simulink model "AariaHIABR2017a"  (R2017a)
settings: Solver=VariableStepAuto  StartTime=0.0  StopTime=inf  FixedStep=0.1  RelTol=1e-3  EnableMultiTasking=on
model workspace (MATLAB code in the model file):
  | my_a =1;
undefined symbols (not defined in the file or in its folder): AARIAENV, AARIAMAN, AARIASEN, Camera, sensor, Source_TS, X, Y, Z
libraries: sm_lib x347, nesl_utility x194, dspmathops x74, simulink x72, vrlib x2, powerlib_meascontrol x1, aerolibanimutils x1, aerolibutil x1
(part 6 of 9)

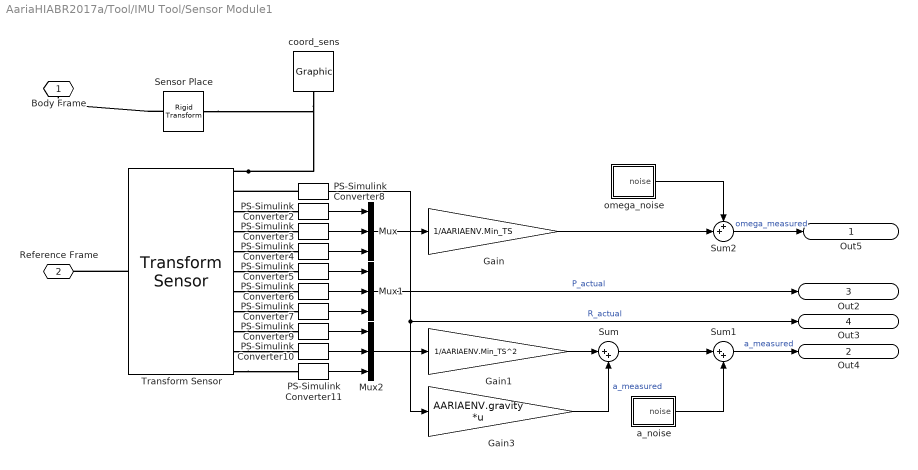
== system AariaHIABR2017a/Tool/IMU Tool/Sensor Module1 ==
  Gain : Gain  Gain=1/AARIAENV.Min_TS
  Gain1 : Gain  Gain=1/AARIAENV.Min_TS^2
  Gain3 : Gain  Gain=AARIAENV.gravity  Multiplication=Matrix(K*u)
  Mux : Mux  Inputs=3
  Mux1 : Mux  Inputs=3
  Mux2 : Mux  Inputs=3
  PS-Simulink Converter{5..11} (7 alike) : nesl_utility/PS-Simulink Converter  PhysicalDomain=network_engine_domain  SubClassName=ps_output  LeftPortType=input  RightPortType=output  PseudoPeriodic=off  Frequencies=[]  Unit=1  AffineConversion=off
  PS-Simulink Converter2 : nesl_utility/PS-Simulink Converter  PhysicalDomain=network_engine_domain  SubClassName=ps_output  LeftPortType=input  RightPortType=output  PseudoPeriodic=off  Frequencies=[]  Unit=rad/s  AffineConversion=off
  PS-Simulink Converter3 : nesl_utility/PS-Simulink Converter  PhysicalDomain=network_engine_domain  SubClassName=ps_output  LeftPortType=input  RightPortType=output  PseudoPeriodic=off  Frequencies=[]  Unit=rad/s  AffineConversion=off
  PS-Simulink Converter4 : nesl_utility/PS-Simulink Converter  PhysicalDomain=network_engine_domain  SubClassName=ps_output  LeftPortType=input  RightPortType=output  PseudoPeriodic=off  Frequencies=[]  Unit=rad/s  AffineConversion=off
  Sensor Place : sm_lib/Frames and Transforms/Rigid Transform  TranslationMethod=Cartesian  TranslationStandardOffset=0  TranslationLengthUnit=m  TranslationStandardAxis=+Z  TranslationCartesianOffset=AARIAMAN.L(nL).S(nS).pose_p  TranslationROffset=0  TranslationROffsetUnits=m  TranslationZOffset=0  TranslationZOffsetUnits=m  TranslationThetaOffset=0  TranslationThetaOffsetUnits=deg  RotationMethod=RotationMatrix  RotationAngleUnits=deg  RotationStandardAxis=+Z  RotationAngle=0.0  RotationArbitraryAxis=[0 0 1]  FollAlignAxisA=+X  BaseAlignAxisA=+Y  FollAlignAxisB=+Y  BaseAlignAxisB=+Z  RotationSequenceAxes=FollowerAxes  RotationSequence=XYX  RotationSequenceAngles=[0 0 0]  RotationSequenceAnglesUnits=deg  RotationMatrix=AARIAMAN.L(nL).S(nS).pose_r
  Sum : Sum  Inputs=|++
  Sum1 : Sum  Inputs=|++
  Sum2 : Sum  Inputs=++|
  Transform Sensor : sm_lib/Frames and Transforms/Transform Sensor  MeasurementFrame=Follower  SenseAngle=off  SenseAxis=off  SenseAngle1=off  SenseAngle2=off  SenseAngle3=off  SenseQ=off  SenseR=on  SenseOmegaX=on  SenseOmegaY=on  SenseOmegaZ=on  SenseOmega1=off  SenseOmega2=off  SenseOmega3=off  SenseQDot=off  SenseRDot=off  SenseAlphaX=off  SenseAlphaY=off  SenseAlphaZ=off  SenseAlpha1=off  SenseAlpha2=off  SenseAlpha3=off  SenseQDDot=off  SenseRDDot=off  SenseX=on  SenseY=on  SenseZ=on  SenseRad=off  SenseAzim=off  SenseDist=off  SenseInc=off  SenseXDot=off  SenseYDot=off  SenseZDot=off  SenseRadDot=off  SenseAzimDot=off  SenseDistDot=off  SenseIncDot=off  SenseXDDot=on  SenseYDDot=on  SenseZDDot=on  SenseRadDDot=off  SenseAzimDDot=off  SenseDistDDot=off  SenseIncDDot=off
  a_noise : Subsystem
  coord_sens : sm_lib/Body Elements/Graphic  GraphicType=Marker  MarkerShape=Frame  MarkerSize=AARIAMAN.vis.coord_sizeS  GraphicVisPropType=SimpleVisualProperties  GraphicDiffuseColor=AARIAMAN.vis.col_s  GraphicSpecularColor=[0.5 0.5 0.5 1.0]  GraphicAmbientColor=[0.15 0.15 0.15 1.0]  GraphicEmissiveColor=[0.0 0.0 0.0 1.0]  GraphicShininess=75  GraphicOpacity=AARIAMAN.vis.opacity_s
      settings: SourceProductName=Simscape Multibody
  omega_noise : Subsystem
  Body Frame : PMIOPort  Port=1  Side=Left
  Reference Frame : PMIOPort  Port=2  Side=Left
  Out5 : Outport
  Out4 : Outport  Port=2
  Out2 : Outport  Port=3
  Out3 : Outport  Port=4
  wires:
  Sum2/1 -> Out5/1  "omega_measured"
  Sum/1 -> Sum1/1
  PS-Simulink Converter8/1 -> Gain3/1, Out3/1  "R_actual"
  Mux2/1 -> Gain1/1
  PS-Simulink Converter7/1 -> Mux1/3
  PS-Simulink Converter5/1 -> Mux1/1
  PS-Simulink Converter6/1 -> Mux1/2
  Mux/1 -> Gain/1
  PS-Simulink Converter4/1 -> Mux/3
  PS-Simulink Converter2/1 -> Mux/1
  PS-Simulink Converter3/1 -> Mux/2
  PS-Simulink Converter9/1 -> Mux2/1
  PS-Simulink Converter11/1 -> Mux2/3
  Mux1/1 -> Out2/1  "P_actual"
  PS-Simulink Converter10/1 -> Mux2/2
  Sum1/1 -> Out4/1  "a_measured"
  Gain3/1 -> Sum/2  "a_measured"
  omega_noise/1(noise) -> Sum2/1
  a_noise/1(noise) -> Sum1/2
  Gain/1 -> Sum2/2
  Gain1/1 -> Sum/1
  connections:
  Transform Sensor/RConn7 -- PS-Simulink Converter6/LConn1
  Transform Sensor/RConn8 -- PS-Simulink Converter7/LConn1
  PS-Simulink Converter8/LConn1 -- Transform Sensor/RConn2
  Transform Sensor/RConn6 -- PS-Simulink Converter5/LConn1
  Transform Sensor/RConn10 -- PS-Simulink Converter10/LConn1
  Transform Sensor/RConn5 -- PS-Simulink Converter4/LConn1
  Transform Sensor/LConn1 -- Reference Frame/RConn1
  Transform Sensor/RConn4 -- PS-Simulink Converter3/LConn1
  Transform Sensor/RConn9 -- PS-Simulink Converter9/LConn1
  Transform Sensor/RConn3 -- PS-Simulink Converter2/LConn1
  Sensor Place/LConn1 -- Body Frame/RConn1
  Transform Sensor/RConn11 -- PS-Simulink Converter11/LConn1
  Transform Sensor/RConn1 -- coord_sens/RConn1 -- Sensor Place/RConn1

== system AariaHIABR2017a/Tool Sensors/Camera sensor/omega_noise ==
  Constant3 : Constant  Value=sensor.gMu
  Constant4 : Constant  Value=sensor.gSigma
  Cumulative Sum : dspmathops/Cumulative Sum  dim=Channels (running sum)  InputProcessing=Columns as channels (frame based)  reset_popup=None  outputDataTypeStr=Inherit: Same as accumulator  outputLastDataTypeStr=Inherit: Same as accumulator  outputMin=[]  outputMax=[]  roundingMode=Floor  overflowMode=off
      settings: SourceProductName=DSP System Toolbox
  Gain1 : Gain  Gain=sensor.ErrorGain
  Mux5 : Mux  Inputs=3
  Normally_distributed_random : MATLAB Function  TreatAsAtomicUnit=on
  Sum3 : Sum  Inputs=+++
  gyro in-run bias : simulink/Sources/Ramp  slope=sensor.gBias  start=0  X0=sensor.gInitBias
  gyro random walk : UniformRandomNumber  Minimum=-sensor.gWalk  Maximum=sensor.gWalk  Seed=sensor.gWalkSeed  SampleTime=Source_TS
  noise : Outport
  wires:
  gyro random walk/1 -> Cumulative Sum/1
  Normally_distributed_random/1(y) -> Sum3/2
  Cumulative Sum/1 -> Sum3/3
  Mux5/1 -> noise/1
  Constant4/1 -> Normally_distributed_random/2(sigma)
  Gain1/1 -> Mux5/3, Mux5/1, Mux5/2
  gyro in-run bias/1 -> Sum3/1
  Sum3/1 -> Gain1/1
  Constant3/1 -> Normally_distributed_random/1(mu)

== system AariaHIABR2017a/Tool Sensors/Camera sensor/placeholder noise 3 ==
  Mux : Mux  Inputs=3
  Uniform Random Number : UniformRandomNumber  Minimum=-0.01  Maximum=0.01  SampleTime=0.1
  noise : Outport
  wires:
  Mux/1 -> noise/1
  Uniform Random Number/1 -> Mux/3, Mux/1, Mux/2

== system AariaHIABR2017a/Tool Sensors/Camera sensor/placeholder noise1 ==
  Mux : Mux  Inputs=3
  Uniform Random Number : UniformRandomNumber  Minimum=-0.01  Maximum=0.01  SampleTime=0.1
  noise : Outport
  wires:
  Uniform Random Number/1 -> Mux/2, Mux/1, Mux/3
  Mux/1 -> noise/1

== system AariaHIABR2017a/Tool Sensors/Camera sensor/placeholder noise2 ==
  Constant : Constant  Value=[1 1 1; 1 1 1; 1 1 1]
  Product : Product
  Uniform Random Number : UniformRandomNumber  Minimum=-0.01  Maximum=0.01  SampleTime=0.1
  noise : Outport
  wires:
  Uniform Random Number/1 -> Product/2
  Product/1 -> noise/1
  Constant/1 -> Product/1

== system AariaHIABR2017a/Tool Sensors/Object tracker/Subsystem ==
  Camera rotation : Inport
  Object rotation : Inport  Port=2
  Matrix Multiply : Product  Multiplication=Matrix(*)
  Object world pose : Outport
  wires:
  Object rotation/1 -> Matrix Multiply/2
  Camera rotation/1 -> Matrix Multiply/1
  Matrix Multiply/1 -> Object world pose/1

== system AariaHIABR2017a/Tool Sensors/Object tracker/placeholder noise1 ==
  Uniform Random Number : UniformRandomNumber  Minimum=-0.1  Maximum=0.1  Seed=1  SampleTime=0.1
  noise : Outport
  wires:
  Uniform Random Number/1 -> noise/1

== system AariaHIABR2017a/Tool Sensors/Object tracker/placeholder noise2 ==
  Uniform Random Number : UniformRandomNumber  Minimum=-0.1  Maximum=0.1  Seed=2  SampleTime=0.1
  noise : Outport
  wires:
  Uniform Random Number/1 -> noise/1

== system AariaHIABR2017a/Tool Sensors/Object tracker/placeholder noise3 ==
  Uniform Random Number : UniformRandomNumber  Minimum=-0.1  Maximum=0.1  SampleTime=0.1
  noise : Outport
  wires:
  Uniform Random Number/1 -> noise/1

== system AariaHIABR2017a/Tool Sensors/Tool sensor1/omega_noise ==
  Constant3 : Constant  Value=sensor.gMu
  Constant4 : Constant  Value=sensor.gSigma
  Cumulative Sum : dspmathops/Cumulative Sum  dim=Channels (running sum)  InputProcessing=Columns as channels (frame based)  reset_popup=None  outputDataTypeStr=Inherit: Same as accumulator  outputLastDataTypeStr=Inherit: Same as accumulator  outputMin=[]  outputMax=[]  roundingMode=Floor  overflowMode=off
      settings: SourceProductName=DSP System Toolbox
  Gain1 : Gain  Gain=sensor.ErrorGain
  Mux5 : Mux  Inputs=3
  Normally_distributed_random : MATLAB Function  TreatAsAtomicUnit=on
  Sum3 : Sum  Inputs=+++
  gyro in-run bias : simulink/Sources/Ramp  slope=sensor.gBias  start=0  X0=sensor.gInitBias
  gyro random walk : UniformRandomNumber  Minimum=-sensor.gWalk  Maximum=sensor.gWalk  Seed=sensor.gWalkSeed  SampleTime=Source_TS
  noise : Outport
  wires:
  gyro random walk/1 -> Cumulative Sum/1
  Normally_distributed_random/1(y) -> Sum3/2
  Cumulative Sum/1 -> Sum3/3
  Mux5/1 -> noise/1
  Constant4/1 -> Normally_distributed_random/2(sigma)
  Gain1/1 -> Mux5/3, Mux5/1, Mux5/2
  gyro in-run bias/1 -> Sum3/1
  Sum3/1 -> Gain1/1
  Constant3/1 -> Normally_distributed_random/1(mu)

== system AariaHIABR2017a/Tool Sensors/Tool sensor1/placeholder noise 3 ==
  Mux : Mux  Inputs=3
  Uniform Random Number : UniformRandomNumber  Minimum=-0.01  Maximum=0.01  SampleTime=0.1
  noise : Outport
  wires:
  Mux/1 -> noise/1
  Uniform Random Number/1 -> Mux/3, Mux/1, Mux/2

== system AariaHIABR2017a/Tool Sensors/Tool sensor1/placeholder noise1 ==
  Mux : Mux  Inputs=3
  Uniform Random Number : UniformRandomNumber  Minimum=-0.01  Maximum=0.01  SampleTime=0.1
  noise : Outport
  wires:
  Uniform Random Number/1 -> Mux/2, Mux/1, Mux/3
  Mux/1 -> noise/1

== system AariaHIABR2017a/Tool Sensors/Tool sensor1/placeholder noise2 ==
  Constant : Constant  Value=[1 1 1; 1 1 1; 1 1 1]
  Product : Product
  Uniform Random Number : UniformRandomNumber  Minimum=-0.01  Maximum=0.01  SampleTime=0.1
  noise : Outport
  wires:
  Uniform Random Number/1 -> Product/2
  Product/1 -> noise/1
  Constant/1 -> Product/1

== system AariaHIABR2017a/Tool Sensors/Tool sensor2/placeholder noise 3 ==
  Mux : Mux  Inputs=3
  Uniform Random Number : UniformRandomNumber  Minimum=-0.01  Maximum=0.01  SampleTime=0.1
  noise : Outport
  wires:
  Uniform Random Number/1 -> Mux/2, Mux/1, Mux/3
  Mux/1 -> noise/1

== system AariaHIABR2017a/Tool Sensors/Tool sensor2/placeholder noise1 ==
  Mux : Mux  Inputs=3
  Uniform Random Number : UniformRandomNumber  Minimum=-0.01  Maximum=0.01  SampleTime=0.1
  noise : Outport
  wires:
  Mux/1 -> noise/1
  Uniform Random Number/1 -> Mux/3, Mux/1, Mux/2

== system AariaHIABR2017a/Tool Sensors/Tool sensor2/placeholder noise2 ==
  Constant : Constant  Value=[1 1 1; 1 1 1; 1 1 1]
  Product : Product
  Uniform Random Number : UniformRandomNumber  Minimum=-0.01  Maximum=0.01  SampleTime=0.1
  noise : Outport
  wires:
  Constant/1 -> Product/1
  Product/1 -> noise/1
  Uniform Random Number/1 -> Product/2

== system AariaHIABR2017a/Base/BaseVSS/BaseEmpty/IMU Base ==
  Sensor Module1 : Subsystem  mask{nL=nL, nS=1}
      mask prompts: nL "Link Number"; nS "Sensor ID of that link"
      mask DialogControl DescGroupVar Prompt: Virtual IMU
      mask DialogControl DescTextVar Prompt: Measures Connected Body's acceleration and angular velocity in the given point
      mask DialogControl Control2 Prompt: The following numbers defines the corresponding numbers for this sensor to read from the parameters file
  Body Coord : PMIOPort  Port=1  Side=Left
  Reference Coord : PMIOPort  Port=2  Side=Left
  Out1 : Outport
  Out2 : Outport  Port=2
  Out3 : Outport  Port=3
  Out4 : Outport  Port=4
  wires:
  Sensor Module1/3(Out2) -> Out3/1
  Sensor Module1/2(Out4) -> Out2/1
  Sensor Module1/4(Out3) -> Out4/1
  Sensor Module1/1(Out5) -> Out1/1
  connections:
  Sensor Module1/LConn2 -- Reference Coord/RConn1
  Sensor Module1/LConn1 -- Body Coord/RConn1

== system AariaHIABR2017a/Base/BaseVSS/BaseMotion/IMU Base ==
  Sensor Module1 : Subsystem  mask{nL=nL, nS=1}
      mask prompts: nL "Link Number"; nS "Sensor ID of that link"
      mask DialogControl DescGroupVar Prompt: Virtual IMU
      mask DialogControl DescTextVar Prompt: Measures Connected Body's acceleration and angular velocity in the given point
      mask DialogControl Control2 Prompt: The following numbers defines the corresponding numbers for this sensor to read from the parameters file
  Body Coord : PMIOPort  Port=1  Side=Left
  Reference Coord : PMIOPort  Port=2  Side=Left
  Out1 : Outport
  Out2 : Outport  Port=2
  Out3 : Outport  Port=3
  Out4 : Outport  Port=4
  wires:
  Sensor Module1/3(Out2) -> Out3/1
  Sensor Module1/2(Out4) -> Out2/1
  Sensor Module1/4(Out3) -> Out4/1
  Sensor Module1/1(Out5) -> Out1/1
  connections:
  Sensor Module1/LConn2 -- Reference Coord/RConn1
  Sensor Module1/LConn1 -- Body Coord/RConn1

== system AariaHIABR2017a/Base/BaseVSS/BaseMotion/x 2motion2 ==
  X : Inport
  Difference : simulink/Discrete/Difference  ICPrevInput=1  InputProcessing=Inherited  OutMin=[]  OutMax=[]  OutDataType=fixdt(1, 16)  OutScaling=2^-10  DoSatur=off
  Difference1 : simulink/Discrete/Difference  ICPrevInput=0  InputProcessing=Inherited  OutMin=[]  OutMax=[]  OutDataType=fixdt(1, 16)  OutScaling=2^-10  DoSatur=off
  Simulink-PS Converter : nesl_utility/Simulink-PS Converter  PhysicalDomain=network_engine_domain  SubClassName=ps_input  LeftPortType=input  RightPortType=output  PseudoPeriodic=off  Frequencies=[]  NoiseDistribution=none  NoiseParameters=[]  Unit=1  AffineConversion=off  FilteringAndDerivatives=provide  SimscapeFilterOrder=1  InputFilterTimeConstant=0.001  UdotUserProvided=2
  Motion for PS : PMIOPort  Port=1  Side=Right
  wires:
  X/1 -> Simulink-PS Converter/1, Difference1/1
  Difference/1 -> Simulink-PS Converter/3
  Difference1/1 -> Difference/1, Simulink-PS Converter/2
  connections:
  Simulink-PS Converter/RConn1 -- Motion for PS/RConn1

== system AariaHIABR2017a/Base/BaseVSS/BaseMotion/x 2motion3 ==
  X : Inport
  Difference : simulink/Discrete/Difference  ICPrevInput=1  InputProcessing=Inherited  OutMin=[]  OutMax=[]  OutDataType=fixdt(1, 16)  OutScaling=2^-10  DoSatur=off
  Difference1 : simulink/Discrete/Difference  ICPrevInput=0  InputProcessing=Inherited  OutMin=[]  OutMax=[]  OutDataType=fixdt(1, 16)  OutScaling=2^-10  DoSatur=off
  Simulink-PS Converter : nesl_utility/Simulink-PS Converter  PhysicalDomain=network_engine_domain  SubClassName=ps_input  LeftPortType=input  RightPortType=output  PseudoPeriodic=off  Frequencies=[]  NoiseDistribution=none  NoiseParameters=[]  Unit=1  AffineConversion=off  FilteringAndDerivatives=provide  SimscapeFilterOrder=1  InputFilterTimeConstant=0.001  UdotUserProvided=2
  Motion for PS : PMIOPort  Port=1  Side=Right
  wires:
  Difference1/1 -> Simulink-PS Converter/2, Difference/1
  Difference/1 -> Simulink-PS Converter/3
  X/1 -> Difference1/1, Simulink-PS Converter/1
  connections:
  Simulink-PS Converter/RConn1 -- Motion for PS/RConn1

== system AariaHIABR2017a/Base/BaseVSS/BaseMotion/x 2motion4 ==
  X : Inport
  Difference : simulink/Discrete/Difference  ICPrevInput=1  InputProcessing=Inherited  OutMin=[]  OutMax=[]  OutDataType=fixdt(1, 16)  OutScaling=2^-10  DoSatur=off
  Difference1 : simulink/Discrete/Difference  ICPrevInput=0  InputProcessing=Inherited  OutMin=[]  OutMax=[]  OutDataType=fixdt(1, 16)  OutScaling=2^-10  DoSatur=off
  Simulink-PS Converter : nesl_utility/Simulink-PS Converter  PhysicalDomain=network_engine_domain  SubClassName=ps_input  LeftPortType=input  RightPortType=output  PseudoPeriodic=off  Frequencies=[]  NoiseDistribution=none  NoiseParameters=[]  Unit=1  AffineConversion=off  FilteringAndDerivatives=provide  SimscapeFilterOrder=1  InputFilterTimeConstant=0.001  UdotUserProvided=2
  Motion for PS : PMIOPort  Port=1  Side=Right
  wires:
  X/1 -> Simulink-PS Converter/1, Difference1/1
  Difference/1 -> Simulink-PS Converter/3
  Difference1/1 -> Difference/1, Simulink-PS Converter/2
  connections:
  Simulink-PS Converter/RConn1 -- Motion for PS/RConn1

== system AariaHIABR2017a/Base/BaseVSS/BaseMotion/x 2motion5 ==
  X : Inport
  Difference : simulink/Discrete/Difference  ICPrevInput=1  InputProcessing=Inherited  OutMin=[]  OutMax=[]  OutDataType=fixdt(1, 16)  OutScaling=2^-10  DoSatur=off
  Difference1 : simulink/Discrete/Difference  ICPrevInput=0  InputProcessing=Inherited  OutMin=[]  OutMax=[]  OutDataType=fixdt(1, 16)  OutScaling=2^-10  DoSatur=off
  Simulink-PS Converter : nesl_utility/Simulink-PS Converter  PhysicalDomain=network_engine_domain  SubClassName=ps_input  LeftPortType=input  RightPortType=output  PseudoPeriodic=off  Frequencies=[]  NoiseDistribution=none  NoiseParameters=[]  Unit=1  AffineConversion=off  FilteringAndDerivatives=provide  SimscapeFilterOrder=1  InputFilterTimeConstant=0.001  UdotUserProvided=2
  Motion for PS : PMIOPort  Port=1  Side=Right
  wires:
  Difference1/1 -> Simulink-PS Converter/2, Difference/1
  Difference/1 -> Simulink-PS Converter/3
  X/1 -> Difference1/1, Simulink-PS Converter/1
  connections:
  Simulink-PS Converter/RConn1 -- Motion for PS/RConn1

== system AariaHIABR2017a/Base/BaseVSS/BaseMotion/x 2motion6 ==
  X : Inport
  Difference : simulink/Discrete/Difference  ICPrevInput=1  InputProcessing=Inherited  OutMin=[]  OutMax=[]  OutDataType=fixdt(1, 16)  OutScaling=2^-10  DoSatur=off
  Difference1 : simulink/Discrete/Difference  ICPrevInput=0  InputProcessing=Inherited  OutMin=[]  OutMax=[]  OutDataType=fixdt(1, 16)  OutScaling=2^-10  DoSatur=off
  Simulink-PS Converter : nesl_utility/Simulink-PS Converter  PhysicalDomain=network_engine_domain  SubClassName=ps_input  LeftPortType=input  RightPortType=output  PseudoPeriodic=off  Frequencies=[]  NoiseDistribution=none  NoiseParameters=[]  Unit=1  AffineConversion=off  FilteringAndDerivatives=provide  SimscapeFilterOrder=1  InputFilterTimeConstant=0.001  UdotUserProvided=2
  Motion for PS : PMIOPort  Port=1  Side=Right
  wires:
  X/1 -> Simulink-PS Converter/1, Difference1/1
  Difference/1 -> Simulink-PS Converter/3
  Difference1/1 -> Difference/1, Simulink-PS Converter/2
  connections:
  Simulink-PS Converter/RConn1 -- Motion for PS/RConn1

== system AariaHIABR2017a/Base/BaseVSS/BaseMotion/x 2motion7 ==
  X : Inport
  Difference : simulink/Discrete/Difference  ICPrevInput=1  InputProcessing=Inherited  OutMin=[]  OutMax=[]  OutDataType=fixdt(1, 16)  OutScaling=2^-10  DoSatur=off
  Difference1 : simulink/Discrete/Difference  ICPrevInput=0  InputProcessing=Inherited  OutMin=[]  OutMax=[]  OutDataType=fixdt(1, 16)  OutScaling=2^-10  DoSatur=off
  Simulink-PS Converter : nesl_utility/Simulink-PS Converter  PhysicalDomain=network_engine_domain  SubClassName=ps_input  LeftPortType=input  RightPortType=output  PseudoPeriodic=off  Frequencies=[]  NoiseDistribution=none  NoiseParameters=[]  Unit=1  AffineConversion=off  FilteringAndDerivatives=provide  SimscapeFilterOrder=1  InputFilterTimeConstant=0.001  UdotUserProvided=2
  Motion for PS : PMIOPort  Port=1  Side=Right
  wires:
  Difference1/1 -> Simulink-PS Converter/2, Difference/1
  Difference/1 -> Simulink-PS Converter/3
  X/1 -> Difference1/1, Simulink-PS Converter/1
  connections:
  Simulink-PS Converter/RConn1 -- Motion for PS/RConn1

== system AariaHIABR2017a/Base/BaseVSS/BaseTorque/IMU Base ==
  Sensor Module1 : Subsystem  mask{nL=nL, nS=1}
      mask prompts: nL "Link Number"; nS "Sensor ID of that link"
      mask DialogControl DescGroupVar Prompt: Virtual IMU
      mask DialogControl DescTextVar Prompt: Measures Connected Body's acceleration and angular velocity in the given point
      mask DialogControl Control2 Prompt: The following numbers defines the corresponding numbers for this sensor to read from the parameters file
  Body Coord : PMIOPort  Port=1  Side=Left
  Reference Coord : PMIOPort  Port=2  Side=Left
  Out1 : Outport
  Out2 : Outport  Port=2
  Out3 : Outport  Port=3
  Out4 : Outport  Port=4
  wires:
  Sensor Module1/3(Out2) -> Out3/1
  Sensor Module1/2(Out4) -> Out2/1
  Sensor Module1/4(Out3) -> Out4/1
  Sensor Module1/1(Out5) -> Out1/1
  connections:
  Sensor Module1/LConn2 -- Reference Coord/RConn1
  Sensor Module1/LConn1 -- Body Coord/RConn1

== system AariaHIABR2017a/Base/BaseVSS/BaseTorque/x 2motion2 ==
  X : Inport
  Difference : simulink/Discrete/Difference  ICPrevInput=1  InputProcessing=Inherited  OutMin=[]  OutMax=[]  OutDataType=fixdt(1, 16)  OutScaling=2^-10  DoSatur=off
  Difference1 : simulink/Discrete/Difference  ICPrevInput=0  InputProcessing=Inherited  OutMin=[]  OutMax=[]  OutDataType=fixdt(1, 16)  OutScaling=2^-10  DoSatur=off
  Simulink-PS Converter : nesl_utility/Simulink-PS Converter  PhysicalDomain=network_engine_domain  SubClassName=ps_input  LeftPortType=input  RightPortType=output  PseudoPeriodic=off  Frequencies=[]  NoiseDistribution=none  NoiseParameters=[]  Unit=1  AffineConversion=off  FilteringAndDerivatives=provide  SimscapeFilterOrder=1  InputFilterTimeConstant=0.001  UdotUserProvided=2
  Motion for PS : PMIOPort  Port=1  Side=Right
  wires:
  X/1 -> Simulink-PS Converter/1, Difference1/1
  Difference/1 -> Simulink-PS Converter/3
  Difference1/1 -> Difference/1, Simulink-PS Converter/2
  connections:
  Simulink-PS Converter/RConn1 -- Motion for PS/RConn1

== system AariaHIABR2017a/Base/BaseVSS/BaseTorque/x 2motion3 ==
  X : Inport
  Difference : simulink/Discrete/Difference  ICPrevInput=1  InputProcessing=Inherited  OutMin=[]  OutMax=[]  OutDataType=fixdt(1, 16)  OutScaling=2^-10  DoSatur=off
  Difference1 : simulink/Discrete/Difference  ICPrevInput=0  InputProcessing=Inherited  OutMin=[]  OutMax=[]  OutDataType=fixdt(1, 16)  OutScaling=2^-10  DoSatur=off
  Simulink-PS Converter : nesl_utility/Simulink-PS Converter  PhysicalDomain=network_engine_domain  SubClassName=ps_input  LeftPortType=input  RightPortType=output  PseudoPeriodic=off  Frequencies=[]  NoiseDistribution=none  NoiseParameters=[]  Unit=1  AffineConversion=off  FilteringAndDerivatives=provide  SimscapeFilterOrder=1  InputFilterTimeConstant=0.001  UdotUserProvided=2
  Motion for PS : PMIOPort  Port=1  Side=Right
  wires:
  Difference1/1 -> Simulink-PS Converter/2, Difference/1
  Difference/1 -> Simulink-PS Converter/3
  X/1 -> Difference1/1, Simulink-PS Converter/1
  connections:
  Simulink-PS Converter/RConn1 -- Motion for PS/RConn1

== system AariaHIABR2017a/Base/BaseVSS/BaseTorque/x 2motion4 ==
  X : Inport
  Difference : simulink/Discrete/Difference  ICPrevInput=1  InputProcessing=Inherited  OutMin=[]  OutMax=[]  OutDataType=fixdt(1, 16)  OutScaling=2^-10  DoSatur=off
  Difference1 : simulink/Discrete/Difference  ICPrevInput=0  InputProcessing=Inherited  OutMin=[]  OutMax=[]  OutDataType=fixdt(1, 16)  OutScaling=2^-10  DoSatur=off
  Simulink-PS Converter : nesl_utility/Simulink-PS Converter  PhysicalDomain=network_engine_domain  SubClassName=ps_input  LeftPortType=input  RightPortType=output  PseudoPeriodic=off  Frequencies=[]  NoiseDistribution=none  NoiseParameters=[]  Unit=1  AffineConversion=off  FilteringAndDerivatives=provide  SimscapeFilterOrder=1  InputFilterTimeConstant=0.001  UdotUserProvided=2
  Motion for PS : PMIOPort  Port=1  Side=Right
  wires:
  X/1 -> Simulink-PS Converter/1, Difference1/1
  Difference/1 -> Simulink-PS Converter/3
  Difference1/1 -> Difference/1, Simulink-PS Converter/2
  connections:
  Simulink-PS Converter/RConn1 -- Motion for PS/RConn1

== system AariaHIABR2017a/Base/BaseVSS/BaseTorque/x 2motion5 ==
  X : Inport
  Difference : simulink/Discrete/Difference  ICPrevInput=1  InputProcessing=Inherited  OutMin=[]  OutMax=[]  OutDataType=fixdt(1, 16)  OutScaling=2^-10  DoSatur=off
  Difference1 : simulink/Discrete/Difference  ICPrevInput=0  InputProcessing=Inherited  OutMin=[]  OutMax=[]  OutDataType=fixdt(1, 16)  OutScaling=2^-10  DoSatur=off
  Simulink-PS Converter : nesl_utility/Simulink-PS Converter  PhysicalDomain=network_engine_domain  SubClassName=ps_input  LeftPortType=input  RightPortType=output  PseudoPeriodic=off  Frequencies=[]  NoiseDistribution=none  NoiseParameters=[]  Unit=1  AffineConversion=off  FilteringAndDerivatives=provide  SimscapeFilterOrder=1  InputFilterTimeConstant=0.001  UdotUserProvided=2
  Motion for PS : PMIOPort  Port=1  Side=Right
  wires:
  Difference1/1 -> Simulink-PS Converter/2, Difference/1
  Difference/1 -> Simulink-PS Converter/3
  X/1 -> Difference1/1, Simulink-PS Converter/1
  connections:
  Simulink-PS Converter/RConn1 -- Motion for PS/RConn1

== system AariaHIABR2017a/Base/BaseVSS/BaseTorque/x 2motion6 ==
  X : Inport
  Difference : simulink/Discrete/Difference  ICPrevInput=1  InputProcessing=Inherited  OutMin=[]  OutMax=[]  OutDataType=fixdt(1, 16)  OutScaling=2^-10  DoSatur=off
  Difference1 : simulink/Discrete/Difference  ICPrevInput=0  InputProcessing=Inherited  OutMin=[]  OutMax=[]  OutDataType=fixdt(1, 16)  OutScaling=2^-10  DoSatur=off
  Simulink-PS Converter : nesl_utility/Simulink-PS Converter  PhysicalDomain=network_engine_domain  SubClassName=ps_input  LeftPortType=input  RightPortType=output  PseudoPeriodic=off  Frequencies=[]  NoiseDistribution=none  NoiseParameters=[]  Unit=1  AffineConversion=off  FilteringAndDerivatives=provide  SimscapeFilterOrder=1  InputFilterTimeConstant=0.001  UdotUserProvided=2
  Motion for PS : PMIOPort  Port=1  Side=Right
  wires:
  X/1 -> Simulink-PS Converter/1, Difference1/1
  Difference/1 -> Simulink-PS Converter/3
  Difference1/1 -> Difference/1, Simulink-PS Converter/2
  connections:
  Simulink-PS Converter/RConn1 -- Motion for PS/RConn1

== system AariaHIABR2017a/Base/BaseVSS/BaseTorque/x 2motion7 ==
  X : Inport
  Difference : simulink/Discrete/Difference  ICPrevInput=1  InputProcessing=Inherited  OutMin=[]  OutMax=[]  OutDataType=fixdt(1, 16)  OutScaling=2^-10  DoSatur=off
  Difference1 : simulink/Discrete/Difference  ICPrevInput=0  InputProcessing=Inherited  OutMin=[]  OutMax=[]  OutDataType=fixdt(1, 16)  OutScaling=2^-10  DoSatur=off
  Simulink-PS Converter : nesl_utility/Simulink-PS Converter  PhysicalDomain=network_engine_domain  SubClassName=ps_input  LeftPortType=input  RightPortType=output  PseudoPeriodic=off  Frequencies=[]  NoiseDistribution=none  NoiseParameters=[]  Unit=1  AffineConversion=off  FilteringAndDerivatives=provide  SimscapeFilterOrder=1  InputFilterTimeConstant=0.001  UdotUserProvided=2
  Motion for PS : PMIOPort  Port=1  Side=Right
  wires:
  Difference1/1 -> Simulink-PS Converter/2, Difference/1
  Difference/1 -> Simulink-PS Converter/3
  X/1 -> Difference1/1, Simulink-PS Converter/1
  connections:
  Simulink-PS Converter/RConn1 -- Motion for PS/RConn1

== system AariaHIABR2017a/Joint1/RevoluteMotion/IMU Sensors/Sensor Module1 ==
  Gain : Gain  Gain=1/AARIAENV.Min_TS
  Gain1 : Gain  Gain=1/AARIAENV.Min_TS^2
  Gain3 : Gain  Gain=AARIAENV.gravity  Multiplication=Matrix(K*u)
  Mux : Mux  Inputs=3
  Mux1 : Mux  Inputs=3
  Mux2 : Mux  Inputs=3
  PS-Simulink Converter{5..11} (7 alike) : nesl_utility/PS-Simulink Converter  PhysicalDomain=network_engine_domain  SubClassName=ps_output  LeftPortType=input  RightPortType=output  PseudoPeriodic=off  Frequencies=[]  Unit=1  AffineConversion=off
  PS-Simulink Converter2 : nesl_utility/PS-Simulink Converter  PhysicalDomain=network_engine_domain  SubClassName=ps_output  LeftPortType=input  RightPortType=output  PseudoPeriodic=off  Frequencies=[]  Unit=rad/s  AffineConversion=off
  PS-Simulink Converter3 : nesl_utility/PS-Simulink Converter  PhysicalDomain=network_engine_domain  SubClassName=ps_output  LeftPortType=input  RightPortType=output  PseudoPeriodic=off  Frequencies=[]  Unit=rad/s  AffineConversion=off
  PS-Simulink Converter4 : nesl_utility/PS-Simulink Converter  PhysicalDomain=network_engine_domain  SubClassName=ps_output  LeftPortType=input  RightPortType=output  PseudoPeriodic=off  Frequencies=[]  Unit=rad/s  AffineConversion=off
  Sensor Place : sm_lib/Frames and Transforms/Rigid Transform  TranslationMethod=Cartesian  TranslationStandardOffset=0  TranslationLengthUnit=m  TranslationStandardAxis=+Z  TranslationCartesianOffset=AARIAMAN.L(nL).S(nS).pose_p  TranslationROffset=0  TranslationROffsetUnits=m  TranslationZOffset=0  TranslationZOffsetUnits=m  TranslationThetaOffset=0  TranslationThetaOffsetUnits=deg  RotationMethod=RotationMatrix  RotationAngleUnits=deg  RotationStandardAxis=+Z  RotationAngle=0.0  RotationArbitraryAxis=[0 0 1]  FollAlignAxisA=+X  BaseAlignAxisA=+Y  FollAlignAxisB=+Y  BaseAlignAxisB=+Z  RotationSequenceAxes=FollowerAxes  RotationSequence=XYX  RotationSequenceAngles=[0 0 0]  RotationSequenceAnglesUnits=deg  RotationMatrix=AARIAMAN.L(nL).S(nS).pose_r
  Sum : Sum  Inputs=|++
  Sum1 : Sum  Inputs=|++
  Sum2 : Sum  Inputs=++|
  Transform Sensor : sm_lib/Frames and Transforms/Transform Sensor  MeasurementFrame=Follower  SenseAngle=off  SenseAxis=off  SenseAngle1=off  SenseAngle2=off  SenseAngle3=off  SenseQ=off  SenseR=on  SenseOmegaX=on  SenseOmegaY=on  SenseOmegaZ=on  SenseOmega1=off  SenseOmega2=off  SenseOmega3=off  SenseQDot=off  SenseRDot=off  SenseAlphaX=off  SenseAlphaY=off  SenseAlphaZ=off  SenseAlpha1=off  SenseAlpha2=off  SenseAlpha3=off  SenseQDDot=off  SenseRDDot=off  SenseX=on  SenseY=on  SenseZ=on  SenseRad=off  SenseAzim=off  SenseDist=off  SenseInc=off  SenseXDot=off  SenseYDot=off  SenseZDot=off  SenseRadDot=off  SenseAzimDot=off  SenseDistDot=off  SenseIncDot=off  SenseXDDot=on  SenseYDDot=on  SenseZDDot=on  SenseRadDDot=off  SenseAzimDDot=off  SenseDistDDot=off  SenseIncDDot=off
  a_noise : Subsystem
  coord_sens : sm_lib/Body Elements/Graphic  GraphicType=Marker  MarkerShape=Frame  MarkerSize=AARIAMAN.vis.coord_sizeS  GraphicVisPropType=SimpleVisualProperties  GraphicDiffuseColor=AARIAMAN.vis.col_s  GraphicSpecularColor=[0.5 0.5 0.5 1.0]  GraphicAmbientColor=[0.15 0.15 0.15 1.0]  GraphicEmissiveColor=[0.0 0.0 0.0 1.0]  GraphicShininess=75  GraphicOpacity=AARIAMAN.vis.opacity_s
      settings: SourceProductName=Simscape Multibody
  omega_noise : Subsystem
  Body Frame : PMIOPort  Port=1  Side=Left
  Reference Frame : PMIOPort  Port=2  Side=Left
  Out5 : Outport
  Out4 : Outport  Port=2
  Out2 : Outport  Port=3
  Out3 : Outport  Port=4
  wires:
  Sum2/1 -> Out5/1  "omega_measured"
  Sum/1 -> Sum1/1
  PS-Simulink Converter8/1 -> Gain3/1, Out3/1  "R_actual"
  Mux2/1 -> Gain1/1
  PS-Simulink Converter7/1 -> Mux1/3
  PS-Simulink Converter5/1 -> Mux1/1
  PS-Simulink Converter6/1 -> Mux1/2
  Mux/1 -> Gain/1
  PS-Simulink Converter4/1 -> Mux/3
  PS-Simulink Converter2/1 -> Mux/1
  PS-Simulink Converter3/1 -> Mux/2
  PS-Simulink Converter9/1 -> Mux2/1
  PS-Simulink Converter11/1 -> Mux2/3
  Mux1/1 -> Out2/1  "P_actual"
  PS-Simulink Converter10/1 -> Mux2/2
  Sum1/1 -> Out4/1  "a_measured"
  Gain3/1 -> Sum/2  "a_measured"
  omega_noise/1(noise) -> Sum2/1
  a_noise/1(noise) -> Sum1/2
  Gain/1 -> Sum2/2
  Gain1/1 -> Sum/1
  connections:
  Transform Sensor/RConn7 -- PS-Simulink Converter6/LConn1
  Transform Sensor/RConn8 -- PS-Simulink Converter7/LConn1
  PS-Simulink Converter8/LConn1 -- Transform Sensor/RConn2
  Transform Sensor/RConn6 -- PS-Simulink Converter5/LConn1
  Transform Sensor/RConn10 -- PS-Simulink Converter10/LConn1
  Transform Sensor/RConn5 -- PS-Simulink Converter4/LConn1
  Transform Sensor/LConn1 -- Reference Frame/RConn1
  Transform Sensor/RConn4 -- PS-Simulink Converter3/LConn1
  Transform Sensor/RConn9 -- PS-Simulink Converter9/LConn1
  Transform Sensor/RConn3 -- PS-Simulink Converter2/LConn1
  Sensor Place/LConn1 -- Body Frame/RConn1
  Transform Sensor/RConn11 -- PS-Simulink Converter11/LConn1
  Transform Sensor/RConn1 -- coord_sens/RConn1 -- Sensor Place/RConn1

== system AariaHIABR2017a/Joint1/RevoluteMotion/IMU Sensors/Sensor Module2 ==
  Gain : Gain  Gain=1/AARIAENV.Min_TS
  Gain1 : Gain  Gain=1/AARIAENV.Min_TS^2
  Gain3 : Gain  Gain=AARIAENV.gravity  Multiplication=Matrix(K*u)
  Mux : Mux  Inputs=3
  Mux1 : Mux  Inputs=3
  Mux2 : Mux  Inputs=3
  PS-Simulink Converter{5..11} (7 alike) : nesl_utility/PS-Simulink Converter  PhysicalDomain=network_engine_domain  SubClassName=ps_output  LeftPortType=input  RightPortType=output  PseudoPeriodic=off  Frequencies=[]  Unit=1  AffineConversion=off
  PS-Simulink Converter2 : nesl_utility/PS-Simulink Converter  PhysicalDomain=network_engine_domain  SubClassName=ps_output  LeftPortType=input  RightPortType=output  PseudoPeriodic=off  Frequencies=[]  Unit=rad/s  AffineConversion=off
  PS-Simulink Converter3 : nesl_utility/PS-Simulink Converter  PhysicalDomain=network_engine_domain  SubClassName=ps_output  LeftPortType=input  RightPortType=output  PseudoPeriodic=off  Frequencies=[]  Unit=rad/s  AffineConversion=off
  PS-Simulink Converter4 : nesl_utility/PS-Simulink Converter  PhysicalDomain=network_engine_domain  SubClassName=ps_output  LeftPortType=input  RightPortType=output  PseudoPeriodic=off  Frequencies=[]  Unit=rad/s  AffineConversion=off
  Sensor Place : sm_lib/Frames and Transforms/Rigid Transform  TranslationMethod=Cartesian  TranslationStandardOffset=0  TranslationLengthUnit=m  TranslationStandardAxis=+Z  TranslationCartesianOffset=AARIAMAN.L(nL).S(nS).pose_p  TranslationROffset=0  TranslationROffsetUnits=m  TranslationZOffset=0  TranslationZOffsetUnits=m  TranslationThetaOffset=0  TranslationThetaOffsetUnits=deg  RotationMethod=RotationMatrix  RotationAngleUnits=deg  RotationStandardAxis=+Z  RotationAngle=0.0  RotationArbitraryAxis=[0 0 1]  FollAlignAxisA=+X  BaseAlignAxisA=+Y  FollAlignAxisB=+Y  BaseAlignAxisB=+Z  RotationSequenceAxes=FollowerAxes  RotationSequence=XYX  RotationSequenceAngles=[0 0 0]  RotationSequenceAnglesUnits=deg  RotationMatrix=AARIAMAN.L(nL).S(nS).pose_r
  Sum : Sum  Inputs=|++
  Sum1 : Sum  Inputs=|++
  Sum2 : Sum  Inputs=++|
  Transform Sensor : sm_lib/Frames and Transforms/Transform Sensor  MeasurementFrame=Follower  SenseAngle=off  SenseAxis=off  SenseAngle1=off  SenseAngle2=off  SenseAngle3=off  SenseQ=off  SenseR=on  SenseOmegaX=on  SenseOmegaY=on  SenseOmegaZ=on  SenseOmega1=off  SenseOmega2=off  SenseOmega3=off  SenseQDot=off  SenseRDot=off  SenseAlphaX=off  SenseAlphaY=off  SenseAlphaZ=off  SenseAlpha1=off  SenseAlpha2=off  SenseAlpha3=off  SenseQDDot=off  SenseRDDot=off  SenseX=on  SenseY=on  SenseZ=on  SenseRad=off  SenseAzim=off  SenseDist=off  SenseInc=off  SenseXDot=off  SenseYDot=off  SenseZDot=off  SenseRadDot=off  SenseAzimDot=off  SenseDistDot=off  SenseIncDot=off  SenseXDDot=on  SenseYDDot=on  SenseZDDot=on  SenseRadDDot=off  SenseAzimDDot=off  SenseDistDDot=off  SenseIncDDot=off
  a_noise : Subsystem
  coord_sens : sm_lib/Body Elements/Graphic  GraphicType=Marker  MarkerShape=Frame  MarkerSize=AARIAMAN.vis.coord_sizeS  GraphicVisPropType=SimpleVisualProperties  GraphicDiffuseColor=AARIAMAN.vis.col_s  GraphicSpecularColor=[0.5 0.5 0.5 1.0]  GraphicAmbientColor=[0.15 0.15 0.15 1.0]  GraphicEmissiveColor=[0.0 0.0 0.0 1.0]  GraphicShininess=75  GraphicOpacity=AARIAMAN.vis.opacity_s
      settings: SourceProductName=Simscape Multibody
  omega_noise : Subsystem
  Body Frame : PMIOPort  Port=1  Side=Left
  Reference Frame : PMIOPort  Port=2  Side=Left
  Out5 : Outport
  Out4 : Outport  Port=2
  Out2 : Outport  Port=3
  Out3 : Outport  Port=4
  wires:
  Sum2/1 -> Out5/1  "omega_measured"
  Sum/1 -> Sum1/1
  PS-Simulink Converter8/1 -> Gain3/1, Out3/1  "R_actual"
  Mux2/1 -> Gain1/1
  PS-Simulink Converter7/1 -> Mux1/3
  PS-Simulink Converter5/1 -> Mux1/1
  PS-Simulink Converter6/1 -> Mux1/2
  Mux/1 -> Gain/1
  PS-Simulink Converter4/1 -> Mux/3
  PS-Simulink Converter2/1 -> Mux/1
  PS-Simulink Converter3/1 -> Mux/2
  PS-Simulink Converter9/1 -> Mux2/1
  PS-Simulink Converter11/1 -> Mux2/3
  Mux1/1 -> Out2/1  "P_actual"
  PS-Simulink Converter10/1 -> Mux2/2
  Sum1/1 -> Out4/1  "a_measured"
  Gain3/1 -> Sum/2  "a_measured"
  omega_noise/1(noise) -> Sum2/1
  a_noise/1(noise) -> Sum1/2
  Gain/1 -> Sum2/2
  Gain1/1 -> Sum/1
  connections:
  Transform Sensor/RConn7 -- PS-Simulink Converter6/LConn1
  Transform Sensor/RConn8 -- PS-Simulink Converter7/LConn1
  PS-Simulink Converter8/LConn1 -- Transform Sensor/RConn2
  Transform Sensor/RConn6 -- PS-Simulink Converter5/LConn1
  Transform Sensor/RConn10 -- PS-Simulink Converter10/LConn1
  Transform Sensor/RConn5 -- PS-Simulink Converter4/LConn1
  Transform Sensor/LConn1 -- Reference Frame/RConn1
  Transform Sensor/RConn4 -- PS-Simulink Converter3/LConn1
  Transform Sensor/RConn9 -- PS-Simulink Converter9/LConn1
  Transform Sensor/RConn3 -- PS-Simulink Converter2/LConn1
  Sensor Place/LConn1 -- Body Frame/RConn1
  Transform Sensor/RConn11 -- PS-Simulink Converter11/LConn1
  Transform Sensor/RConn1 -- coord_sens/RConn1 -- Sensor Place/RConn1

== system AariaHIABR2017a/Joint2/RevoluteMotion/IMU Sensors/Sensor Module1 ==
  Gain : Gain  Gain=1/AARIAENV.Min_TS
  Gain1 : Gain  Gain=1/AARIAENV.Min_TS^2
  Gain3 : Gain  Gain=AARIAENV.gravity  Multiplication=Matrix(K*u)
  Mux : Mux  Inputs=3
  Mux1 : Mux  Inputs=3
  Mux2 : Mux  Inputs=3
  PS-Simulink Converter{5..11} (7 alike) : nesl_utility/PS-Simulink Converter  PhysicalDomain=network_engine_domain  SubClassName=ps_output  LeftPortType=input  RightPortType=output  PseudoPeriodic=off  Frequencies=[]  Unit=1  AffineConversion=off
  PS-Simulink Converter2 : nesl_utility/PS-Simulink Converter  PhysicalDomain=network_engine_domain  SubClassName=ps_output  LeftPortType=input  RightPortType=output  PseudoPeriodic=off  Frequencies=[]  Unit=rad/s  AffineConversion=off
  PS-Simulink Converter3 : nesl_utility/PS-Simulink Converter  PhysicalDomain=network_engine_domain  SubClassName=ps_output  LeftPortType=input  RightPortType=output  PseudoPeriodic=off  Frequencies=[]  Unit=rad/s  AffineConversion=off
  PS-Simulink Converter4 : nesl_utility/PS-Simulink Converter  PhysicalDomain=network_engine_domain  SubClassName=ps_output  LeftPortType=input  RightPortType=output  PseudoPeriodic=off  Frequencies=[]  Unit=rad/s  AffineConversion=off
  Sensor Place : sm_lib/Frames and Transforms/Rigid Transform  TranslationMethod=Cartesian  TranslationStandardOffset=0  TranslationLengthUnit=m  TranslationStandardAxis=+Z  TranslationCartesianOffset=AARIAMAN.L(nL).S(nS).pose_p  TranslationROffset=0  TranslationROffsetUnits=m  TranslationZOffset=0  TranslationZOffsetUnits=m  TranslationThetaOffset=0  TranslationThetaOffsetUnits=deg  RotationMethod=RotationMatrix  RotationAngleUnits=deg  RotationStandardAxis=+Z  RotationAngle=0.0  RotationArbitraryAxis=[0 0 1]  FollAlignAxisA=+X  BaseAlignAxisA=+Y  FollAlignAxisB=+Y  BaseAlignAxisB=+Z  RotationSequenceAxes=FollowerAxes  RotationSequence=XYX  RotationSequenceAngles=[0 0 0]  RotationSequenceAnglesUnits=deg  RotationMatrix=AARIAMAN.L(nL).S(nS).pose_r
  Sum : Sum  Inputs=|++
  Sum1 : Sum  Inputs=|++
  Sum2 : Sum  Inputs=++|
  Transform Sensor : sm_lib/Frames and Transforms/Transform Sensor  MeasurementFrame=Follower  SenseAngle=off  SenseAxis=off  SenseAngle1=off  SenseAngle2=off  SenseAngle3=off  SenseQ=off  SenseR=on  SenseOmegaX=on  SenseOmegaY=on  SenseOmegaZ=on  SenseOmega1=off  SenseOmega2=off  SenseOmega3=off  SenseQDot=off  SenseRDot=off  SenseAlphaX=off  SenseAlphaY=off  SenseAlphaZ=off  SenseAlpha1=off  SenseAlpha2=off  SenseAlpha3=off  SenseQDDot=off  SenseRDDot=off  SenseX=on  SenseY=on  SenseZ=on  SenseRad=off  SenseAzim=off  SenseDist=off  SenseInc=off  SenseXDot=off  SenseYDot=off  SenseZDot=off  SenseRadDot=off  SenseAzimDot=off  SenseDistDot=off  SenseIncDot=off  SenseXDDot=on  SenseYDDot=on  SenseZDDot=on  SenseRadDDot=off  SenseAzimDDot=off  SenseDistDDot=off  SenseIncDDot=off
  a_noise : Subsystem
  coord_sens : sm_lib/Body Elements/Graphic  GraphicType=Marker  MarkerShape=Frame  MarkerSize=AARIAMAN.vis.coord_sizeS  GraphicVisPropType=SimpleVisualProperties  GraphicDiffuseColor=AARIAMAN.vis.col_s  GraphicSpecularColor=[0.5 0.5 0.5 1.0]  GraphicAmbientColor=[0.15 0.15 0.15 1.0]  GraphicEmissiveColor=[0.0 0.0 0.0 1.0]  GraphicShininess=75  GraphicOpacity=AARIAMAN.vis.opacity_s
      settings: SourceProductName=Simscape Multibody
  omega_noise : Subsystem
  Body Frame : PMIOPort  Port=1  Side=Left
  Reference Frame : PMIOPort  Port=2  Side=Left
  Out5 : Outport
  Out4 : Outport  Port=2
  Out2 : Outport  Port=3
  Out3 : Outport  Port=4
  wires:
  Sum2/1 -> Out5/1  "omega_measured"
  Sum/1 -> Sum1/1
  PS-Simulink Converter8/1 -> Gain3/1, Out3/1  "R_actual"
  Mux2/1 -> Gain1/1
  PS-Simulink Converter7/1 -> Mux1/3
  PS-Simulink Converter5/1 -> Mux1/1
  PS-Simulink Converter6/1 -> Mux1/2
  Mux/1 -> Gain/1
  PS-Simulink Converter4/1 -> Mux/3
  PS-Simulink Converter2/1 -> Mux/1
  PS-Simulink Converter3/1 -> Mux/2
  PS-Simulink Converter9/1 -> Mux2/1
  PS-Simulink Converter11/1 -> Mux2/3
  Mux1/1 -> Out2/1  "P_actual"
  PS-Simulink Converter10/1 -> Mux2/2
  Sum1/1 -> Out4/1  "a_measured"
  Gain3/1 -> Sum/2  "a_measured"
  omega_noise/1(noise) -> Sum2/1
  a_noise/1(noise) -> Sum1/2
  Gain/1 -> Sum2/2
  Gain1/1 -> Sum/1
  connections:
  Transform Sensor/RConn7 -- PS-Simulink Converter6/LConn1
  Transform Sensor/RConn8 -- PS-Simulink Converter7/LConn1
  PS-Simulink Converter8/LConn1 -- Transform Sensor/RConn2
  Transform Sensor/RConn6 -- PS-Simulink Converter5/LConn1
  Transform Sensor/RConn10 -- PS-Simulink Converter10/LConn1
  Transform Sensor/RConn5 -- PS-Simulink Converter4/LConn1
  Transform Sensor/LConn1 -- Reference Frame/RConn1
  Transform Sensor/RConn4 -- PS-Simulink Converter3/LConn1
  Transform Sensor/RConn9 -- PS-Simulink Converter9/LConn1
  Transform Sensor/RConn3 -- PS-Simulink Converter2/LConn1
  Sensor Place/LConn1 -- Body Frame/RConn1
  Transform Sensor/RConn11 -- PS-Simulink Converter11/LConn1
  Transform Sensor/RConn1 -- coord_sens/RConn1 -- Sensor Place/RConn1

== system AariaHIABR2017a/Joint2/RevoluteMotion/IMU Sensors/Sensor Module2 ==
  Gain : Gain  Gain=1/AARIAENV.Min_TS
  Gain1 : Gain  Gain=1/AARIAENV.Min_TS^2
  Gain3 : Gain  Gain=AARIAENV.gravity  Multiplication=Matrix(K*u)
  Mux : Mux  Inputs=3
  Mux1 : Mux  Inputs=3
  Mux2 : Mux  Inputs=3
  PS-Simulink Converter{5..11} (7 alike) : nesl_utility/PS-Simulink Converter  PhysicalDomain=network_engine_domain  SubClassName=ps_output  LeftPortType=input  RightPortType=output  PseudoPeriodic=off  Frequencies=[]  Unit=1  AffineConversion=off
  PS-Simulink Converter2 : nesl_utility/PS-Simulink Converter  PhysicalDomain=network_engine_domain  SubClassName=ps_output  LeftPortType=input  RightPortType=output  PseudoPeriodic=off  Frequencies=[]  Unit=rad/s  AffineConversion=off
  PS-Simulink Converter3 : nesl_utility/PS-Simulink Converter  PhysicalDomain=network_engine_domain  SubClassName=ps_output  LeftPortType=input  RightPortType=output  PseudoPeriodic=off  Frequencies=[]  Unit=rad/s  AffineConversion=off
  PS-Simulink Converter4 : nesl_utility/PS-Simulink Converter  PhysicalDomain=network_engine_domain  SubClassName=ps_output  LeftPortType=input  RightPortType=output  PseudoPeriodic=off  Frequencies=[]  Unit=rad/s  AffineConversion=off
  Sensor Place : sm_lib/Frames and Transforms/Rigid Transform  TranslationMethod=Cartesian  TranslationStandardOffset=0  TranslationLengthUnit=m  TranslationStandardAxis=+Z  TranslationCartesianOffset=AARIAMAN.L(nL).S(nS).pose_p  TranslationROffset=0  TranslationROffsetUnits=m  TranslationZOffset=0  TranslationZOffsetUnits=m  TranslationThetaOffset=0  TranslationThetaOffsetUnits=deg  RotationMethod=RotationMatrix  RotationAngleUnits=deg  RotationStandardAxis=+Z  RotationAngle=0.0  RotationArbitraryAxis=[0 0 1]  FollAlignAxisA=+X  BaseAlignAxisA=+Y  FollAlignAxisB=+Y  BaseAlignAxisB=+Z  RotationSequenceAxes=FollowerAxes  RotationSequence=XYX  RotationSequenceAngles=[0 0 0]  RotationSequenceAnglesUnits=deg  RotationMatrix=AARIAMAN.L(nL).S(nS).pose_r
  Sum : Sum  Inputs=|++
  Sum1 : Sum  Inputs=|++
  Sum2 : Sum  Inputs=++|
  Transform Sensor : sm_lib/Frames and Transforms/Transform Sensor  MeasurementFrame=Follower  SenseAngle=off  SenseAxis=off  SenseAngle1=off  SenseAngle2=off  SenseAngle3=off  SenseQ=off  SenseR=on  SenseOmegaX=on  SenseOmegaY=on  SenseOmegaZ=on  SenseOmega1=off  SenseOmega2=off  SenseOmega3=off  SenseQDot=off  SenseRDot=off  SenseAlphaX=off  SenseAlphaY=off  SenseAlphaZ=off  SenseAlpha1=off  SenseAlpha2=off  SenseAlpha3=off  SenseQDDot=off  SenseRDDot=off  SenseX=on  SenseY=on  SenseZ=on  SenseRad=off  SenseAzim=off  SenseDist=off  SenseInc=off  SenseXDot=off  SenseYDot=off  SenseZDot=off  SenseRadDot=off  SenseAzimDot=off  SenseDistDot=off  SenseIncDot=off  SenseXDDot=on  SenseYDDot=on  SenseZDDot=on  SenseRadDDot=off  SenseAzimDDot=off  SenseDistDDot=off  SenseIncDDot=off
  a_noise : Subsystem
  coord_sens : sm_lib/Body Elements/Graphic  GraphicType=Marker  MarkerShape=Frame  MarkerSize=AARIAMAN.vis.coord_sizeS  GraphicVisPropType=SimpleVisualProperties  GraphicDiffuseColor=AARIAMAN.vis.col_s  GraphicSpecularColor=[0.5 0.5 0.5 1.0]  GraphicAmbientColor=[0.15 0.15 0.15 1.0]  GraphicEmissiveColor=[0.0 0.0 0.0 1.0]  GraphicShininess=75  GraphicOpacity=AARIAMAN.vis.opacity_s
      settings: SourceProductName=Simscape Multibody
  omega_noise : Subsystem
  Body Frame : PMIOPort  Port=1  Side=Left
  Reference Frame : PMIOPort  Port=2  Side=Left
  Out5 : Outport
  Out4 : Outport  Port=2
  Out2 : Outport  Port=3
  Out3 : Outport  Port=4
  wires:
  Sum2/1 -> Out5/1  "omega_measured"
  Sum/1 -> Sum1/1
  PS-Simulink Converter8/1 -> Gain3/1, Out3/1  "R_actual"
  Mux2/1 -> Gain1/1
  PS-Simulink Converter7/1 -> Mux1/3
  PS-Simulink Converter5/1 -> Mux1/1
  PS-Simulink Converter6/1 -> Mux1/2
  Mux/1 -> Gain/1
  PS-Simulink Converter4/1 -> Mux/3
  PS-Simulink Converter2/1 -> Mux/1
  PS-Simulink Converter3/1 -> Mux/2
  PS-Simulink Converter9/1 -> Mux2/1
  PS-Simulink Converter11/1 -> Mux2/3
  Mux1/1 -> Out2/1  "P_actual"
  PS-Simulink Converter10/1 -> Mux2/2
  Sum1/1 -> Out4/1  "a_measured"
  Gain3/1 -> Sum/2  "a_measured"
  omega_noise/1(noise) -> Sum2/1
  a_noise/1(noise) -> Sum1/2
  Gain/1 -> Sum2/2
  Gain1/1 -> Sum/1
  connections:
  Transform Sensor/RConn7 -- PS-Simulink Converter6/LConn1
  Transform Sensor/RConn8 -- PS-Simulink Converter7/LConn1
  PS-Simulink Converter8/LConn1 -- Transform Sensor/RConn2
  Transform Sensor/RConn6 -- PS-Simulink Converter5/LConn1
  Transform Sensor/RConn10 -- PS-Simulink Converter10/LConn1
  Transform Sensor/RConn5 -- PS-Simulink Converter4/LConn1
  Transform Sensor/LConn1 -- Reference Frame/RConn1
  Transform Sensor/RConn4 -- PS-Simulink Converter3/LConn1
  Transform Sensor/RConn9 -- PS-Simulink Converter9/LConn1
  Transform Sensor/RConn3 -- PS-Simulink Converter2/LConn1
  Sensor Place/LConn1 -- Body Frame/RConn1
  Transform Sensor/RConn11 -- PS-Simulink Converter11/LConn1
  Transform Sensor/RConn1 -- coord_sens/RConn1 -- Sensor Place/RConn1
